simulink library "Plateau_Z_Only"  (R2026a)
settings: Solver=VariableStepAuto
undefined symbols (not defined in the file): Scene
libraries: Scene_Utilities x1
Description:
  | Simscape Vehicle Templates Library
  | 
  | Copyright 2018-2026 The MathWorks, Inc.
settings Model: Creator=smiller  LastModifiedBy=smiller

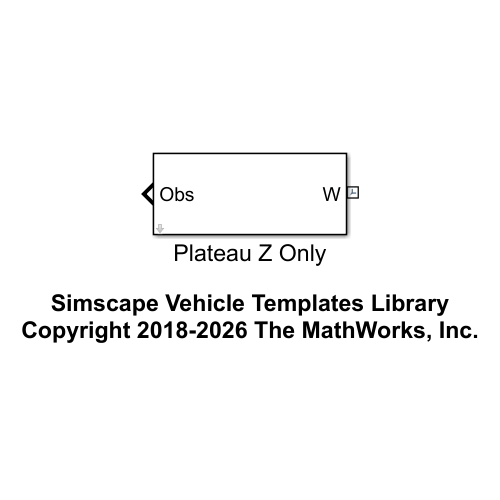
[thumbnail: Simulink's stored preview of the top-level diagram]
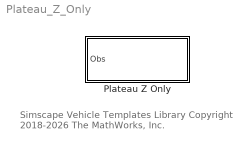
== system Plateau_Z_Only ==
  note: Simscape Vehicle Templates Library
      | Copyright 2018-2026 The MathWorks, Inc.
  Plateau Z Only : Subsystem  VariantControl=Plateau_Z_Only  mask{RDF_Polyline=Scene.RDF_Plateau}
      mask prompts: RDF_Polyline "RDF Polyline (structure)"

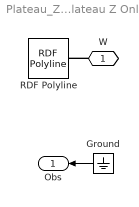
== system Plateau_Z_Only/Plateau Z Only ==
  Ground : Ground
  RDF Polyline : Scene_Utilities/RDF Polyline  road_extr_data_L=RDF_Polyline.Road.extr_data_L  road_extr_data_R=RDF_Polyline.Road.extr_data_R  road_profile_sep=RDF_Polyline.Road.profile_separation  road_w=RDF_Polyline.Road.w  road_x=RDF_Polyline.Road.x  road_z=RDF_Polyline.Road.z  road_yaw=RDF_Polyline.Road.yaw  road_clr=RDF_Polyline.Road.clr  road_opc=RDF_Polyline.Road.opc
  W : PMIOPort  Side=Left
  Obs : Outport  VectorParamsAs1DForOutWhenUnconnected=off
  wires:
  Ground/1 -> Obs/1
  connections:
  W/RConn1 -- RDF Polyline/RConn1
